simulink model "suspensao_modelagem_atualizada"  (R2015a)
settings: Solver=ode23t  StartTime=0.0  StopTime=10.0  RelTol=1e-3
settings Model: Creator=Joacy Mesquita  LastModifiedBy=Joacy Mesquita

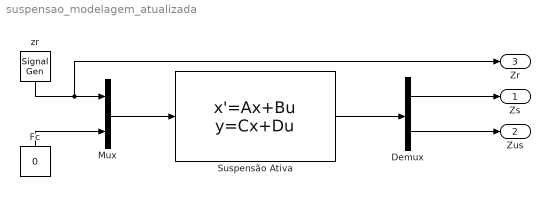
== system suspensao_modelagem_atualizada ==
  Demux : Demux  Outputs=2
  Fc : Constant  Value=0
  Mux : Mux  Inputs=2
  Suspensão Ativa : StateSpace  A=[1 0 0 0; -367.346938775510 -3.06122448979592 367.346938775510 3.06122448979592; 0 0 1 0; 900 7.50000000000000 -2150 -12.5000000000000]  B=[0 0; 0 0.408163265306122; 0 0; 1250 -1]  C=[1 0 0 0; 0 0 1 0]  D=[0 0; 0 0]  X0=0
  zr : SignalGenerator  WaveForm=square  Amplitude=-0.01  Frequency=0.3
  Zs : Outport
  Zus : Outport  Port=2
  Zr : Outport  Port=3
  wires:
  Mux/1 -> Suspensão Ativa/1
  zr/1 -> Zr/1, Mux/1
  Fc/1 -> Mux/2
  Suspensão Ativa/1 -> Demux/1
  Demux/1 -> Zs/1
  Demux/2 -> Zus/1
